simulink model "consensus_demo"  (Simulink 7.4)
settings: Solver=ode45  StartTime=0.0  StopTime=100.0  RelTol=1e-3
settings Model: Creator=francisco  LastModifiedBy=francisco
settings DataIOCC: SaveState=on

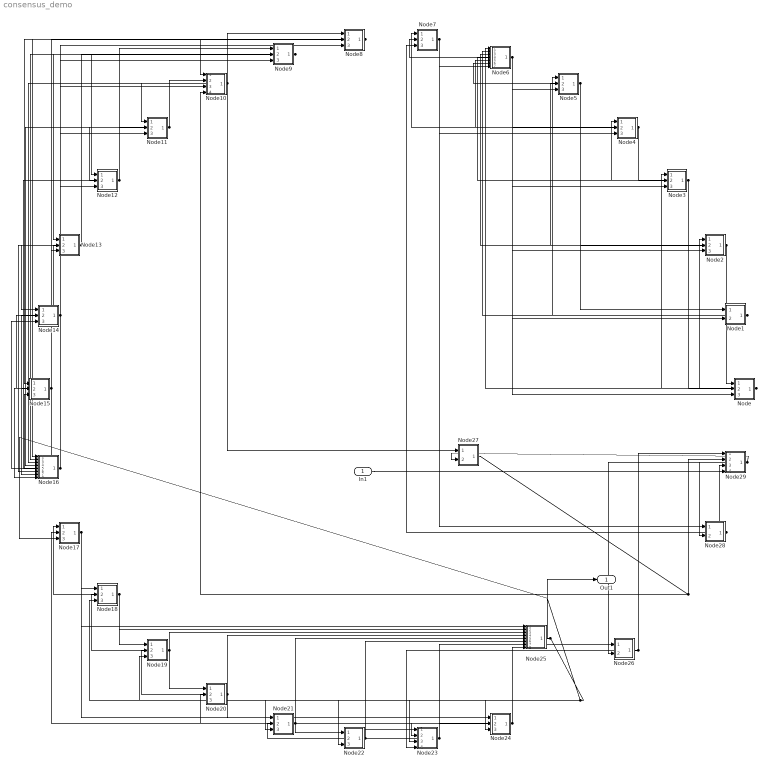
== system consensus_demo ==
  In1 : Inport  OutDataType=fixdt(1, 16)  OutScaling=2^0
  Node : Subsystem
  Node1 : Subsystem
  Node10 : Subsystem
  Node11 : Subsystem
  Node12 : Subsystem
  Node13 : Subsystem
  Node14 : Subsystem
  Node15 : Subsystem
  Node16 : Subsystem
  Node17 : Subsystem
  Node18 : Subsystem
  Node19 : Subsystem
  Node2 : Subsystem
  Node20 : Subsystem
  Node21 : Subsystem
  Node22 : Subsystem
  Node23 : Subsystem
  Node24 : Subsystem
  Node25 : Subsystem
  Node26 : Subsystem
  Node27 : Subsystem
  Node28 : Subsystem
  Node29 : Subsystem
  Node3 : Subsystem
  Node4 : Subsystem
  Node5 : Subsystem
  Node6 : Subsystem
  Node7 : Subsystem
  Node8 : Subsystem
  Node9 : Subsystem
  Out1 : Outport  OutDataType=fixdt(1, 16)  OutScaling=2^0
  wires:
  Node/1(Out1) -> Node2/1(In1), Node3/1(In1), Node6/1(In1)
  Node1/1(Out1) -> Node5/1(In1), Node6/2(In2)
  Node2/1(Out1) -> Node/1(In1), Node5/2(In3), Node6/3(In3)
  Node3/1(Out1) -> Node/2(In4), Node4/1(In1), Node6/4(In4)
  Node4/1(Out1) -> Node3/2(In5), Node6/5(In5), Node7/1(In1)
  Node5/1(Out1) -> Node1/1(In1), Node2/2(In6), Node6/6(In6)
  Node6/1(Out1) -> Node/3(In7), Node1/2(In7), Node2/3(In7), Node3/3(In7), Node4/2(In7), Node5/3(In7), Node7/2(In7)
  Node7/1(Out1) -> Node4/3(In8), Node6/7(In8), Node28/1(In1)
  Node8/1(Out1) -> Node10/1(In1), Node15/1(In1), Node16/1(In1)
  Node9/1(Out1) -> Node12/1(In1), Node13/1(In1), Node16/2(In10)
  Node10/1(Out1) -> Node8/1(In1), Node11/1(In1), Node16/3(In11), Node27/1(In1)
  Node11/1(Out1) -> Node10/2(In12), Node12/2(In12), Node16/4(In12)
  Node12/1(Out1) -> Node9/1(In1), Node11/2(In13), Node16/5(In13)
  Node13/1(Out1) -> Node9/2(In14), Node14/1(In1), Node16/6(In14)
  Node14/1(Out1) -> Node13/2(In15), Node15/2(In15), Node16/7(In15)
  Node15/1(Out1) -> Node8/2(In16), Node14/2(In16), Node16/8(In16)
  Node16/1(Out1) -> Node8/3(In17), Node9/3(In17), Node10/3(In17), Node11/3(In17), Node12/3(In17), Node13/3(In17), Node14/3(In17), Node15/3(In17)
  Node17/1(Out1) -> Node18/1(In1), Node24/1(In1), Node25/1(In1)
  Node18/1(Out1) -> Node17/1(In1), Node19/1(In1), Node25/2(In19)
  Node19/1(Out1) -> Node18/2(In20), Node20/1(In1), Node25/3(In20)
  Node20/1(Out1) -> Node19/2(In21), Node21/1(In1), Node25/4(In21)
  Node21/1(Out1) -> Node20/2(In22), Node22/1(In1), Node25/5(In22)
  Node22/1(Out1) -> Node21/2(In23), Node23/1(In1), Node25/6(In23)
  Node23/1(Out1) -> Node22/2(In24), Node24/2(In24), Node25/7(In24), Node26/1(In1)
  Node24/1(Out1) -> Node17/2(In25), Node23/2(In25), Node25/8(In25)
  Node25/1(Out1) -> Node17/3(In26), Node18/3(In26), Node19/3(In26), Node20/3(In26), Node21/3(In26), Node22/3(In26), Node23/3(In26), Node24/3(In26), Out1/1
  Node26/1(Out1) -> Node23/4(In27), Node29/1(In1)
  Node27/1(Out1) -> Node10/4(In28), Node29/2(In28)
  Node28/1(Out1) -> Node7/3(In29), Node29/3(In29)
  Node29/1(Out1) -> Node26/2(In30), Node27/2(In30), Node28/2(In30)
  In1/1 -> Node29/4(In2)

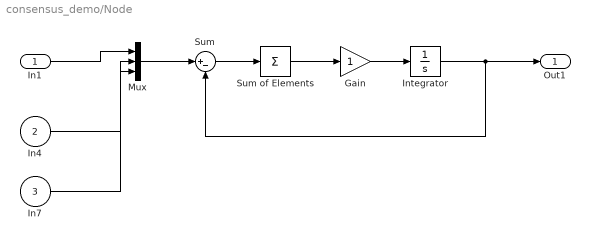
== system consensus_demo/Node ==
  In1 : Inport
  In4 : Inport  Port=2
  In7 : Inport  Port=3
  Gain : Gain  ParameterDataType=fixdt(1, 16)  ParameterScaling=2^0  OutDataType=fixdt(1, 16)  OutScaling=2^0
  Integrator : Integrator  InitialCondition=100*(rand()-0.5)
  Mux : Mux  Inputs=3
  Sum : Sum  Inputs=|+-  OutDataType=fixdt(1, 16)  OutScaling=2^0
  Sum of Elements : Sum  Inputs=+  OutDataType=fixdt(1, 16)  OutScaling=2^-10
  Out1 : Outport
  wires:
  In7/1 -> Mux/3
  In4/1 -> Mux/2
  Integrator/1 -> Sum/2, Out1/1
  Gain/1 -> Integrator/1
  Sum of Elements/1 -> Gain/1
  Sum/1 -> Sum of Elements/1
  Mux/1 -> Sum/1
  In1/1 -> Mux/1

== system consensus_demo/Node1 ==
  In1 : Inport
  In7 : Inport  Port=2
  Gain : Gain  ParameterDataType=fixdt(1, 16)  ParameterScaling=2^0  OutDataType=fixdt(1, 16)  OutScaling=2^0
  Integrator : Integrator  InitialCondition=100*(rand()-0.5)
  Mux : Mux  Inputs=2
  Sum : Sum  Inputs=|+-  OutDataType=fixdt(1, 16)  OutScaling=2^0
  Sum of Elements : Sum  Inputs=+  OutDataType=fixdt(1, 16)  OutScaling=2^-10
  Out1 : Outport
  wires:
  In7/1 -> Mux/2
  Integrator/1 -> Sum/2, Out1/1
  Gain/1 -> Integrator/1
  Sum of Elements/1 -> Gain/1
  Sum/1 -> Sum of Elements/1
  Mux/1 -> Sum/1
  In1/1 -> Mux/1

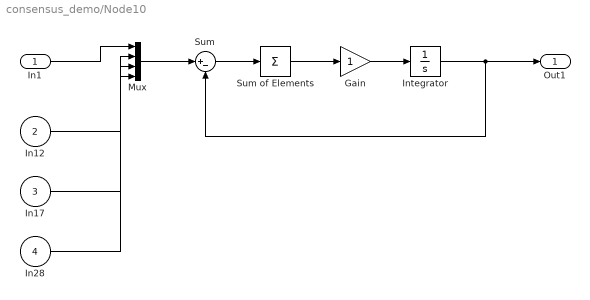
== system consensus_demo/Node10 ==
  In1 : Inport
  In12 : Inport  Port=2
  In17 : Inport  Port=3
  In28 : Inport  Port=4
  Gain : Gain  ParameterDataType=fixdt(1, 16)  ParameterScaling=2^0  OutDataType=fixdt(1, 16)  OutScaling=2^0
  Integrator : Integrator  InitialCondition=100*(rand()-0.5)
  Mux : Mux
  Sum : Sum  Inputs=|+-  OutDataType=fixdt(1, 16)  OutScaling=2^0
  Sum of Elements : Sum  Inputs=+  OutDataType=fixdt(1, 16)  OutScaling=2^-10
  Out1 : Outport
  wires:
  In28/1 -> Mux/4
  In17/1 -> Mux/3
  In12/1 -> Mux/2
  Integrator/1 -> Sum/2, Out1/1
  Gain/1 -> Integrator/1
  Sum of Elements/1 -> Gain/1
  Sum/1 -> Sum of Elements/1
  Mux/1 -> Sum/1
  In1/1 -> Mux/1

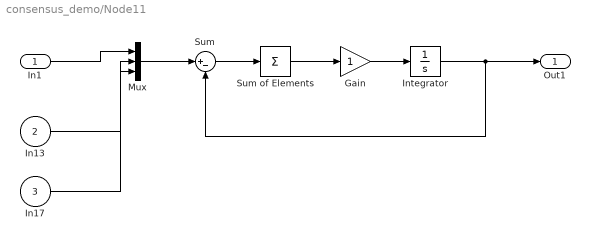
== system consensus_demo/Node11 ==
  In1 : Inport
  In13 : Inport  Port=2
  In17 : Inport  Port=3
  Gain : Gain  ParameterDataType=fixdt(1, 16)  ParameterScaling=2^0  OutDataType=fixdt(1, 16)  OutScaling=2^0
  Integrator : Integrator  InitialCondition=100*(rand()-0.5)
  Mux : Mux  Inputs=3
  Sum : Sum  Inputs=|+-  OutDataType=fixdt(1, 16)  OutScaling=2^0
  Sum of Elements : Sum  Inputs=+  OutDataType=fixdt(1, 16)  OutScaling=2^-10
  Out1 : Outport
  wires:
  In17/1 -> Mux/3
  In13/1 -> Mux/2
  Integrator/1 -> Sum/2, Out1/1
  Gain/1 -> Integrator/1
  Sum of Elements/1 -> Gain/1
  Sum/1 -> Sum of Elements/1
  Mux/1 -> Sum/1
  In1/1 -> Mux/1

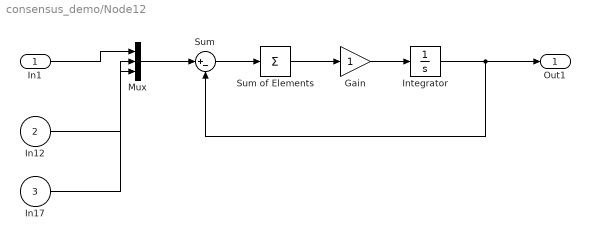
== system consensus_demo/Node12 ==
  In1 : Inport
  In12 : Inport  Port=2
  In17 : Inport  Port=3
  Gain : Gain  ParameterDataType=fixdt(1, 16)  ParameterScaling=2^0  OutDataType=fixdt(1, 16)  OutScaling=2^0
  Integrator : Integrator  InitialCondition=100*(rand()-0.5)
  Mux : Mux  Inputs=3
  Sum : Sum  Inputs=|+-  OutDataType=fixdt(1, 16)  OutScaling=2^0
  Sum of Elements : Sum  Inputs=+  OutDataType=fixdt(1, 16)  OutScaling=2^-10
  Out1 : Outport
  wires:
  In17/1 -> Mux/3
  In12/1 -> Mux/2
  Integrator/1 -> Sum/2, Out1/1
  Gain/1 -> Integrator/1
  Sum of Elements/1 -> Gain/1
  Sum/1 -> Sum of Elements/1
  Mux/1 -> Sum/1
  In1/1 -> Mux/1

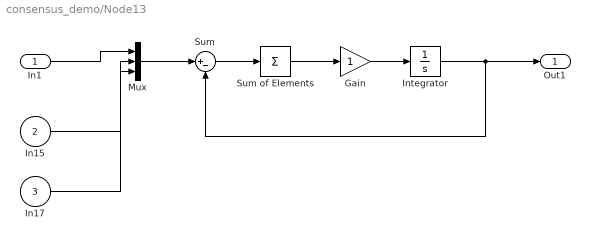
== system consensus_demo/Node13 ==
  In1 : Inport
  In15 : Inport  Port=2
  In17 : Inport  Port=3
  Gain : Gain  ParameterDataType=fixdt(1, 16)  ParameterScaling=2^0  OutDataType=fixdt(1, 16)  OutScaling=2^0
  Integrator : Integrator  InitialCondition=100*(rand()-0.5)
  Mux : Mux  Inputs=3
  Sum : Sum  Inputs=|+-  OutDataType=fixdt(1, 16)  OutScaling=2^0
  Sum of Elements : Sum  Inputs=+  OutDataType=fixdt(1, 16)  OutScaling=2^-10
  Out1 : Outport
  wires:
  In17/1 -> Mux/3
  In15/1 -> Mux/2
  Integrator/1 -> Sum/2, Out1/1
  Gain/1 -> Integrator/1
  Sum of Elements/1 -> Gain/1
  Sum/1 -> Sum of Elements/1
  Mux/1 -> Sum/1
  In1/1 -> Mux/1

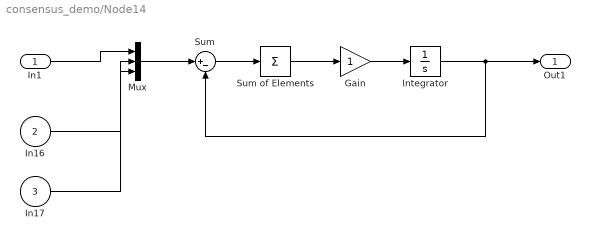
== system consensus_demo/Node14 ==
  In1 : Inport
  In16 : Inport  Port=2
  In17 : Inport  Port=3
  Gain : Gain  ParameterDataType=fixdt(1, 16)  ParameterScaling=2^0  OutDataType=fixdt(1, 16)  OutScaling=2^0
  Integrator : Integrator  InitialCondition=100*(rand()-0.5)
  Mux : Mux  Inputs=3
  Sum : Sum  Inputs=|+-  OutDataType=fixdt(1, 16)  OutScaling=2^0
  Sum of Elements : Sum  Inputs=+  OutDataType=fixdt(1, 16)  OutScaling=2^-10
  Out1 : Outport
  wires:
  In17/1 -> Mux/3
  In16/1 -> Mux/2
  Integrator/1 -> Sum/2, Out1/1
  Gain/1 -> Integrator/1
  Sum of Elements/1 -> Gain/1
  Sum/1 -> Sum of Elements/1
  Mux/1 -> Sum/1
  In1/1 -> Mux/1

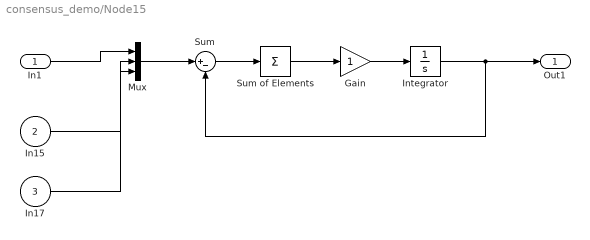
== system consensus_demo/Node15 ==
  In1 : Inport
  In15 : Inport  Port=2
  In17 : Inport  Port=3
  Gain : Gain  ParameterDataType=fixdt(1, 16)  ParameterScaling=2^0  OutDataType=fixdt(1, 16)  OutScaling=2^0
  Integrator : Integrator  InitialCondition=100*(rand()-0.5)
  Mux : Mux  Inputs=3
  Sum : Sum  Inputs=|+-  OutDataType=fixdt(1, 16)  OutScaling=2^0
  Sum of Elements : Sum  Inputs=+  OutDataType=fixdt(1, 16)  OutScaling=2^-10
  Out1 : Outport
  wires:
  In17/1 -> Mux/3
  In15/1 -> Mux/2
  Integrator/1 -> Sum/2, Out1/1
  Gain/1 -> Integrator/1
  Sum of Elements/1 -> Gain/1
  Sum/1 -> Sum of Elements/1
  Mux/1 -> Sum/1
  In1/1 -> Mux/1

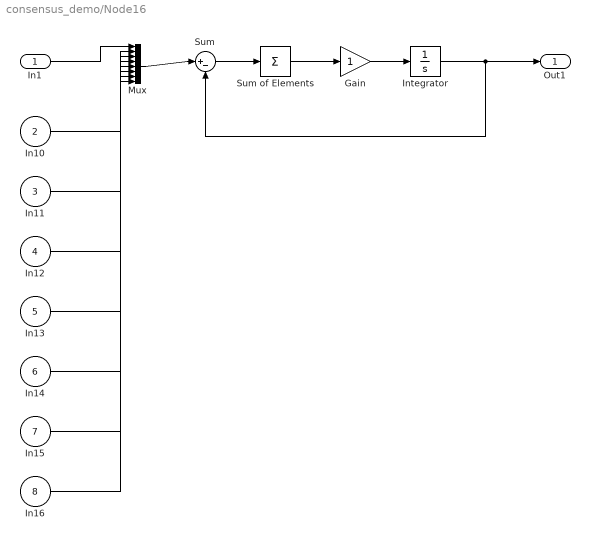
== system consensus_demo/Node16 ==
  In1 : Inport
  In10 : Inport  Port=2
  In11 : Inport  Port=3
  In12 : Inport  Port=4
  In13 : Inport  Port=5
  In14 : Inport  Port=6
  In15 : Inport  Port=7
  In16 : Inport  Port=8
  Gain : Gain  ParameterDataType=fixdt(1, 16)  ParameterScaling=2^0  OutDataType=fixdt(1, 16)  OutScaling=2^0
  Integrator : Integrator  InitialCondition=100*(rand()-0.5)
  Mux : Mux  Inputs=8
  Sum : Sum  Inputs=|+-  OutDataType=fixdt(1, 16)  OutScaling=2^0
  Sum of Elements : Sum  Inputs=+  OutDataType=fixdt(1, 16)  OutScaling=2^-10
  Out1 : Outport
  wires:
  In16/1 -> Mux/8
  In15/1 -> Mux/7
  In14/1 -> Mux/6
  In13/1 -> Mux/5
  In12/1 -> Mux/4
  In11/1 -> Mux/3
  In10/1 -> Mux/2
  Integrator/1 -> Sum/2, Out1/1
  Gain/1 -> Integrator/1
  Sum of Elements/1 -> Gain/1
  Sum/1 -> Sum of Elements/1
  Mux/1 -> Sum/1
  In1/1 -> Mux/1

== system consensus_demo/Node17 ==
  In1 : Inport
  In25 : Inport  Port=2
  In26 : Inport  Port=3
  Gain : Gain  ParameterDataType=fixdt(1, 16)  ParameterScaling=2^0  OutDataType=fixdt(1, 16)  OutScaling=2^0
  Integrator : Integrator  InitialCondition=100*(rand()-0.5)
  Mux : Mux  Inputs=3
  Sum : Sum  Inputs=|+-  OutDataType=fixdt(1, 16)  OutScaling=2^0
  Sum of Elements : Sum  Inputs=+  OutDataType=fixdt(1, 16)  OutScaling=2^-10
  Out1 : Outport
  wires:
  In26/1 -> Mux/3
  In25/1 -> Mux/2
  Integrator/1 -> Sum/2, Out1/1
  Gain/1 -> Integrator/1
  Sum of Elements/1 -> Gain/1
  Sum/1 -> Sum of Elements/1
  Mux/1 -> Sum/1
  In1/1 -> Mux/1

== system consensus_demo/Node18 ==
  In1 : Inport
  In20 : Inport  Port=2
  In26 : Inport  Port=3
  Gain : Gain  ParameterDataType=fixdt(1, 16)  ParameterScaling=2^0  OutDataType=fixdt(1, 16)  OutScaling=2^0
  Integrator : Integrator  InitialCondition=100*(rand()-0.5)
  Mux : Mux  Inputs=3
  Sum : Sum  Inputs=|+-  OutDataType=fixdt(1, 16)  OutScaling=2^0
  Sum of Elements : Sum  Inputs=+  OutDataType=fixdt(1, 16)  OutScaling=2^-10
  Out1 : Outport
  wires:
  In26/1 -> Mux/3
  In20/1 -> Mux/2
  Integrator/1 -> Sum/2, Out1/1
  Gain/1 -> Integrator/1
  Sum of Elements/1 -> Gain/1
  Sum/1 -> Sum of Elements/1
  Mux/1 -> Sum/1
  In1/1 -> Mux/1

== system consensus_demo/Node19 ==
  In1 : Inport
  In21 : Inport  Port=2
  In26 : Inport  Port=3
  Gain : Gain  ParameterDataType=fixdt(1, 16)  ParameterScaling=2^0  OutDataType=fixdt(1, 16)  OutScaling=2^0
  Integrator : Integrator  InitialCondition=100*(rand()-0.5)
  Mux : Mux  Inputs=3
  Sum : Sum  Inputs=|+-  OutDataType=fixdt(1, 16)  OutScaling=2^0
  Sum of Elements : Sum  Inputs=+  OutDataType=fixdt(1, 16)  OutScaling=2^-10
  Out1 : Outport
  wires:
  In26/1 -> Mux/3
  In21/1 -> Mux/2
  Integrator/1 -> Sum/2, Out1/1
  Gain/1 -> Integrator/1
  Sum of Elements/1 -> Gain/1
  Sum/1 -> Sum of Elements/1
  Mux/1 -> Sum/1
  In1/1 -> Mux/1

== system consensus_demo/Node2 ==
  In1 : Inport
  In6 : Inport  Port=2
  In7 : Inport  Port=3
  Gain : Gain  ParameterDataType=fixdt(1, 16)  ParameterScaling=2^0  OutDataType=fixdt(1, 16)  OutScaling=2^0
  Integrator : Integrator  InitialCondition=100*(rand()-0.5)
  Mux : Mux  Inputs=3
  Sum : Sum  Inputs=|+-  OutDataType=fixdt(1, 16)  OutScaling=2^0
  Sum of Elements : Sum  Inputs=+  OutDataType=fixdt(1, 16)  OutScaling=2^-10
  Out1 : Outport
  wires:
  In7/1 -> Mux/3
  In6/1 -> Mux/2
  Integrator/1 -> Sum/2, Out1/1
  Gain/1 -> Integrator/1
  Sum of Elements/1 -> Gain/1
  Sum/1 -> Sum of Elements/1
  Mux/1 -> Sum/1
  In1/1 -> Mux/1

== system consensus_demo/Node20 ==
  In1 : Inport
  In22 : Inport  Port=2
  In26 : Inport  Port=3
  Gain : Gain  ParameterDataType=fixdt(1, 16)  ParameterScaling=2^0  OutDataType=fixdt(1, 16)  OutScaling=2^0
  Integrator : Integrator  InitialCondition=100*(rand()-0.5)
  Mux : Mux  Inputs=3
  Sum : Sum  Inputs=|+-  OutDataType=fixdt(1, 16)  OutScaling=2^0
  Sum of Elements : Sum  Inputs=+  OutDataType=fixdt(1, 16)  OutScaling=2^-10
  Out1 : Outport
  wires:
  In26/1 -> Mux/3
  In22/1 -> Mux/2
  Integrator/1 -> Sum/2, Out1/1
  Gain/1 -> Integrator/1
  Sum of Elements/1 -> Gain/1
  Sum/1 -> Sum of Elements/1
  Mux/1 -> Sum/1
  In1/1 -> Mux/1

== system consensus_demo/Node21 ==
  In1 : Inport
  In23 : Inport  Port=2
  In26 : Inport  Port=3
  Gain : Gain  ParameterDataType=fixdt(1, 16)  ParameterScaling=2^0  OutDataType=fixdt(1, 16)  OutScaling=2^0
  Integrator : Integrator  InitialCondition=100*(rand()-0.5)
  Mux : Mux  Inputs=3
  Sum : Sum  Inputs=|+-  OutDataType=fixdt(1, 16)  OutScaling=2^0
  Sum of Elements : Sum  Inputs=+  OutDataType=fixdt(1, 16)  OutScaling=2^-10
  Out1 : Outport
  wires:
  In26/1 -> Mux/3
  In23/1 -> Mux/2
  Integrator/1 -> Sum/2, Out1/1
  Gain/1 -> Integrator/1
  Sum of Elements/1 -> Gain/1
  Sum/1 -> Sum of Elements/1
  Mux/1 -> Sum/1
  In1/1 -> Mux/1

== system consensus_demo/Node22 ==
  In1 : Inport
  In24 : Inport  Port=2
  In26 : Inport  Port=3
  Gain : Gain  ParameterDataType=fixdt(1, 16)  ParameterScaling=2^0  OutDataType=fixdt(1, 16)  OutScaling=2^0
  Integrator : Integrator  InitialCondition=100*(rand()-0.5)
  Mux : Mux  Inputs=3
  Sum : Sum  Inputs=|+-  OutDataType=fixdt(1, 16)  OutScaling=2^0
  Sum of Elements : Sum  Inputs=+  OutDataType=fixdt(1, 16)  OutScaling=2^-10
  Out1 : Outport
  wires:
  In26/1 -> Mux/3
  In24/1 -> Mux/2
  Integrator/1 -> Sum/2, Out1/1
  Gain/1 -> Integrator/1
  Sum of Elements/1 -> Gain/1
  Sum/1 -> Sum of Elements/1
  Mux/1 -> Sum/1
  In1/1 -> Mux/1

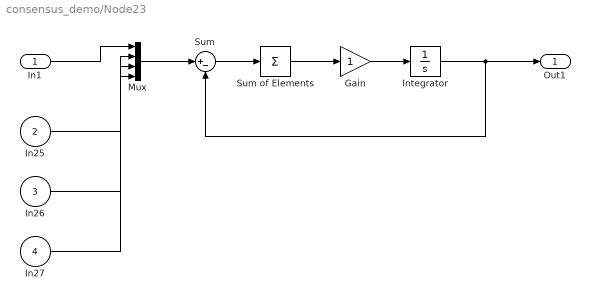
== system consensus_demo/Node23 ==
  In1 : Inport
  In25 : Inport  Port=2
  In26 : Inport  Port=3
  In27 : Inport  Port=4
  Gain : Gain  ParameterDataType=fixdt(1, 16)  ParameterScaling=2^0  OutDataType=fixdt(1, 16)  OutScaling=2^0
  Integrator : Integrator  InitialCondition=100*(rand()-0.5)
  Mux : Mux
  Sum : Sum  Inputs=|+-  OutDataType=fixdt(1, 16)  OutScaling=2^0
  Sum of Elements : Sum  Inputs=+  OutDataType=fixdt(1, 16)  OutScaling=2^-10
  Out1 : Outport
  wires:
  In27/1 -> Mux/4
  In26/1 -> Mux/3
  In25/1 -> Mux/2
  Integrator/1 -> Sum/2, Out1/1
  Gain/1 -> Integrator/1
  Sum of Elements/1 -> Gain/1
  Sum/1 -> Sum of Elements/1
  Mux/1 -> Sum/1
  In1/1 -> Mux/1

== system consensus_demo/Node24 ==
  In1 : Inport
  In24 : Inport  Port=2
  In26 : Inport  Port=3
  Gain : Gain  ParameterDataType=fixdt(1, 16)  ParameterScaling=2^0  OutDataType=fixdt(1, 16)  OutScaling=2^0
  Integrator : Integrator  InitialCondition=100*(rand()-0.5)
  Mux : Mux  Inputs=3
  Sum : Sum  Inputs=|+-  OutDataType=fixdt(1, 16)  OutScaling=2^0
  Sum of Elements : Sum  Inputs=+  OutDataType=fixdt(1, 16)  OutScaling=2^-10
  Out1 : Outport
  wires:
  In26/1 -> Mux/3
  In24/1 -> Mux/2
  Integrator/1 -> Sum/2, Out1/1
  Gain/1 -> Integrator/1
  Sum of Elements/1 -> Gain/1
  Sum/1 -> Sum of Elements/1
  Mux/1 -> Sum/1
  In1/1 -> Mux/1

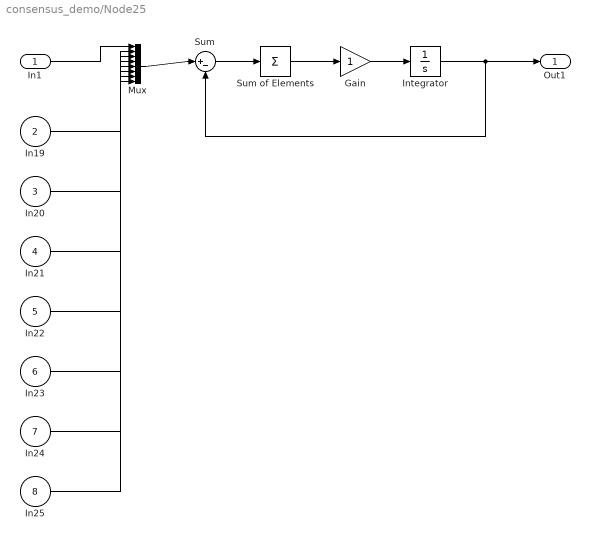
== system consensus_demo/Node25 ==
  In1 : Inport
  In19 : Inport  Port=2
  In20 : Inport  Port=3
  In21 : Inport  Port=4
  In22 : Inport  Port=5
  In23 : Inport  Port=6
  In24 : Inport  Port=7
  In25 : Inport  Port=8
  Gain : Gain  ParameterDataType=fixdt(1, 16)  ParameterScaling=2^0  OutDataType=fixdt(1, 16)  OutScaling=2^0
  Integrator : Integrator  InitialCondition=100*(rand()-0.5)
  Mux : Mux  Inputs=8
  Sum : Sum  Inputs=|+-  OutDataType=fixdt(1, 16)  OutScaling=2^0
  Sum of Elements : Sum  Inputs=+  OutDataType=fixdt(1, 16)  OutScaling=2^-10
  Out1 : Outport
  wires:
  In25/1 -> Mux/8
  In24/1 -> Mux/7
  In23/1 -> Mux/6
  In22/1 -> Mux/5
  In21/1 -> Mux/4
  In20/1 -> Mux/3
  In19/1 -> Mux/2
  Integrator/1 -> Sum/2, Out1/1
  Gain/1 -> Integrator/1
  Sum of Elements/1 -> Gain/1
  Sum/1 -> Sum of Elements/1
  Mux/1 -> Sum/1
  In1/1 -> Mux/1

== system consensus_demo/Node26 ==
  In1 : Inport
  In30 : Inport  Port=2
  Gain : Gain  ParameterDataType=fixdt(1, 16)  ParameterScaling=2^0  OutDataType=fixdt(1, 16)  OutScaling=2^0
  Integrator : Integrator  InitialCondition=100*(rand()-0.5)
  Mux : Mux  Inputs=2
  Sum : Sum  Inputs=|+-  OutDataType=fixdt(1, 16)  OutScaling=2^0
  Sum of Elements : Sum  Inputs=+  OutDataType=fixdt(1, 16)  OutScaling=2^-10
  Out1 : Outport
  wires:
  In30/1 -> Mux/2
  Integrator/1 -> Sum/2, Out1/1
  Gain/1 -> Integrator/1
  Sum of Elements/1 -> Gain/1
  Sum/1 -> Sum of Elements/1
  Mux/1 -> Sum/1
  In1/1 -> Mux/1

== system consensus_demo/Node27 ==
  In1 : Inport
  In30 : Inport  Port=2
  Gain : Gain  ParameterDataType=fixdt(1, 16)  ParameterScaling=2^0  OutDataType=fixdt(1, 16)  OutScaling=2^0
  Integrator : Integrator  InitialCondition=100*(rand()-0.5)
  Mux : Mux  Inputs=2
  Sum : Sum  Inputs=|+-  OutDataType=fixdt(1, 16)  OutScaling=2^0
  Sum of Elements : Sum  Inputs=+  OutDataType=fixdt(1, 16)  OutScaling=2^-10
  Out1 : Outport
  wires:
  In30/1 -> Mux/2
  Integrator/1 -> Sum/2, Out1/1
  Gain/1 -> Integrator/1
  Sum of Elements/1 -> Gain/1
  Sum/1 -> Sum of Elements/1
  Mux/1 -> Sum/1
  In1/1 -> Mux/1

== system consensus_demo/Node28 ==
  In1 : Inport
  In30 : Inport  Port=2
  Gain : Gain  ParameterDataType=fixdt(1, 16)  ParameterScaling=2^0  OutDataType=fixdt(1, 16)  OutScaling=2^0
  Integrator : Integrator  InitialCondition=100*(rand()-0.5)
  Mux : Mux  Inputs=2
  Sum : Sum  Inputs=|+-  OutDataType=fixdt(1, 16)  OutScaling=2^0
  Sum of Elements : Sum  Inputs=+  OutDataType=fixdt(1, 16)  OutScaling=2^-10
  Out1 : Outport
  wires:
  In30/1 -> Mux/2
  Integrator/1 -> Sum/2, Out1/1
  Gain/1 -> Integrator/1
  Sum of Elements/1 -> Gain/1
  Sum/1 -> Sum of Elements/1
  Mux/1 -> Sum/1
  In1/1 -> Mux/1

== system consensus_demo/Node29 ==
  In1 : Inport
  In28 : Inport  Port=2
  In29 : Inport  Port=3
  In2 : Inport  Port=4  OutDataType=fixdt(1, 16)  OutScaling=2^0
  Constant : Constant  Value=0  OutDataType=fixdt(1, 16)  OutScaling=2^0
  Integrator : Integrator  InitialCondition=50*rand()
  Mux : Mux
  Terminator : Terminator
  Out1 : Outport
  wires:
  In29/1 -> Mux/3
  In28/1 -> Mux/2
  Constant/1 -> Integrator/1
  Integrator/1 -> Out1/1
  Mux/1 -> Terminator/1
  In1/1 -> Mux/1
  In2/1 -> Mux/4

== system consensus_demo/Node3 ==
  In1 : Inport
  In5 : Inport  Port=2
  In7 : Inport  Port=3
  Gain : Gain  ParameterDataType=fixdt(1, 16)  ParameterScaling=2^0  OutDataType=fixdt(1, 16)  OutScaling=2^0
  Integrator : Integrator  InitialCondition=100*(rand()-0.5)
  Mux : Mux  Inputs=3
  Sum : Sum  Inputs=|+-  OutDataType=fixdt(1, 16)  OutScaling=2^0
  Sum of Elements : Sum  Inputs=+  OutDataType=fixdt(1, 16)  OutScaling=2^-10
  Out1 : Outport
  wires:
  In7/1 -> Mux/3
  In5/1 -> Mux/2
  Integrator/1 -> Sum/2, Out1/1
  Gain/1 -> Integrator/1
  Sum of Elements/1 -> Gain/1
  Sum/1 -> Sum of Elements/1
  Mux/1 -> Sum/1
  In1/1 -> Mux/1

== system consensus_demo/Node4 ==
  In1 : Inport
  In7 : Inport  Port=2
  In8 : Inport  Port=3
  Gain : Gain  ParameterDataType=fixdt(1, 16)  ParameterScaling=2^0  OutDataType=fixdt(1, 16)  OutScaling=2^0
  Integrator : Integrator  InitialCondition=100*(rand()-0.5)
  Mux : Mux  Inputs=3
  Sum : Sum  Inputs=|+-  OutDataType=fixdt(1, 16)  OutScaling=2^0
  Sum of Elements : Sum  Inputs=+  OutDataType=fixdt(1, 16)  OutScaling=2^-10
  Out1 : Outport
  wires:
  In8/1 -> Mux/3
  In7/1 -> Mux/2
  Integrator/1 -> Sum/2, Out1/1
  Gain/1 -> Integrator/1
  Sum of Elements/1 -> Gain/1
  Sum/1 -> Sum of Elements/1
  Mux/1 -> Sum/1
  In1/1 -> Mux/1

== system consensus_demo/Node5 ==
  In1 : Inport
  In3 : Inport  Port=2
  In7 : Inport  Port=3
  Gain : Gain  ParameterDataType=fixdt(1, 16)  ParameterScaling=2^0  OutDataType=fixdt(1, 16)  OutScaling=2^0
  Integrator : Integrator  InitialCondition=100*(rand()-0.5)
  Mux : Mux  Inputs=3
  Sum : Sum  Inputs=|+-  OutDataType=fixdt(1, 16)  OutScaling=2^0
  Sum of Elements : Sum  Inputs=+  OutDataType=fixdt(1, 16)  OutScaling=2^-10
  Out1 : Outport
  wires:
  In7/1 -> Mux/3
  In3/1 -> Mux/2
  Integrator/1 -> Sum/2, Out1/1
  Gain/1 -> Integrator/1
  Sum of Elements/1 -> Gain/1
  Sum/1 -> Sum of Elements/1
  Mux/1 -> Sum/1
  In1/1 -> Mux/1

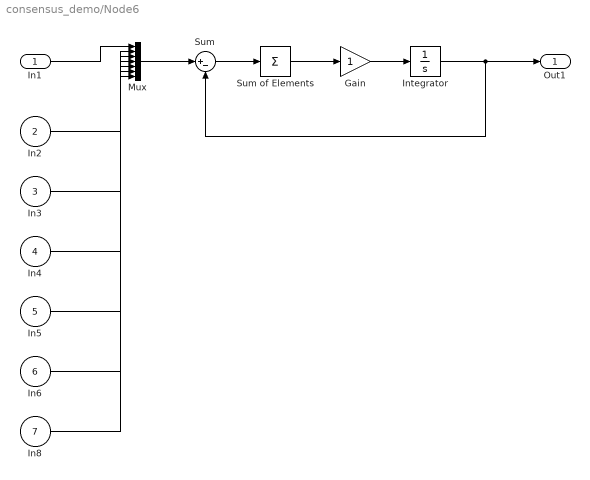
== system consensus_demo/Node6 ==
  In1 : Inport
  In2 : Inport  Port=2
  In3 : Inport  Port=3
  In4 : Inport  Port=4
  In5 : Inport  Port=5
  In6 : Inport  Port=6
  In8 : Inport  Port=7
  Gain : Gain  ParameterDataType=fixdt(1, 16)  ParameterScaling=2^0  OutDataType=fixdt(1, 16)  OutScaling=2^0
  Integrator : Integrator  InitialCondition=100*(rand()-0.5)
  Mux : Mux  Inputs=7
  Sum : Sum  Inputs=|+-  OutDataType=fixdt(1, 16)  OutScaling=2^0
  Sum of Elements : Sum  Inputs=+  OutDataType=fixdt(1, 16)  OutScaling=2^-10
  Out1 : Outport
  wires:
  In8/1 -> Mux/7
  In6/1 -> Mux/6
  In5/1 -> Mux/5
  In4/1 -> Mux/4
  In3/1 -> Mux/3
  In2/1 -> Mux/2
  Integrator/1 -> Sum/2, Out1/1
  Gain/1 -> Integrator/1
  Sum of Elements/1 -> Gain/1
  Sum/1 -> Sum of Elements/1
  Mux/1 -> Sum/1
  In1/1 -> Mux/1

== system consensus_demo/Node7 ==
  In1 : Inport
  In7 : Inport  Port=2
  In29 : Inport  Port=3
  Gain : Gain  ParameterDataType=fixdt(1, 16)  ParameterScaling=2^0  OutDataType=fixdt(1, 16)  OutScaling=2^0
  Integrator : Integrator  InitialCondition=100*(rand()-0.5)
  Mux : Mux  Inputs=3
  Sum : Sum  Inputs=|+-  OutDataType=fixdt(1, 16)  OutScaling=2^0
  Sum of Elements : Sum  Inputs=+  OutDataType=fixdt(1, 16)  OutScaling=2^-10
  Out1 : Outport
  wires:
  In29/1 -> Mux/3
  In7/1 -> Mux/2
  Integrator/1 -> Sum/2, Out1/1
  Gain/1 -> Integrator/1
  Sum of Elements/1 -> Gain/1
  Sum/1 -> Sum of Elements/1
  Mux/1 -> Sum/1
  In1/1 -> Mux/1

== system consensus_demo/Node8 ==
  In1 : Inport
  In16 : Inport  Port=2
  In17 : Inport  Port=3
  Gain : Gain  ParameterDataType=fixdt(1, 16)  ParameterScaling=2^0  OutDataType=fixdt(1, 16)  OutScaling=2^0
  Integrator : Integrator  InitialCondition=100*(rand()-0.5)
  Mux : Mux  Inputs=3
  Sum : Sum  Inputs=|+-  OutDataType=fixdt(1, 16)  OutScaling=2^0
  Sum of Elements : Sum  Inputs=+  OutDataType=fixdt(1, 16)  OutScaling=2^-10
  Out1 : Outport
  wires:
  In17/1 -> Mux/3
  In16/1 -> Mux/2
  Integrator/1 -> Sum/2, Out1/1
  Gain/1 -> Integrator/1
  Sum of Elements/1 -> Gain/1
  Sum/1 -> Sum of Elements/1
  Mux/1 -> Sum/1
  In1/1 -> Mux/1

== system consensus_demo/Node9 ==
  In1 : Inport
  In14 : Inport  Port=2
  In17 : Inport  Port=3
  Gain : Gain  ParameterDataType=fixdt(1, 16)  ParameterScaling=2^0  OutDataType=fixdt(1, 16)  OutScaling=2^0
  Integrator : Integrator  InitialCondition=100*(rand()-0.5)
  Mux : Mux  Inputs=3
  Sum : Sum  Inputs=|+-  OutDataType=fixdt(1, 16)  OutScaling=2^0
  Sum of Elements : Sum  Inputs=+  OutDataType=fixdt(1, 16)  OutScaling=2^-10
  Out1 : Outport
  wires:
  In17/1 -> Mux/3
  In14/1 -> Mux/2
  Integrator/1 -> Sum/2, Out1/1
  Gain/1 -> Integrator/1
  Sum of Elements/1 -> Gain/1
  Sum/1 -> Sum of Elements/1
  Mux/1 -> Sum/1
  In1/1 -> Mux/1
